simulink model "ball_and_plate_discreto2"  (Simulink 8.7)
settings: Solver=ode3  StartTime=0.0  StopTime=200  FixedStep=0.05  RelTol=1e-3
undefined symbols (not defined in the file): Newton, Raphson
settings Model: Creator=mario  LastModifiedBy=mario
settings DataIOCC: SaveFormat=Structure  SignalLoggingSaveFormat=ModelDataLogs
settings OptimizationCC: ExpressionDepthLimit=2147483647
settings DebuggingCC: SolverPrmCheckMsg=warning  FcnCallInpInsideContextMsg=UseLocalSettings  StateNameClashWarn=warning
settings GRTTargetCC: CombineOutputUpdateFcns=off  GRTInterface=on

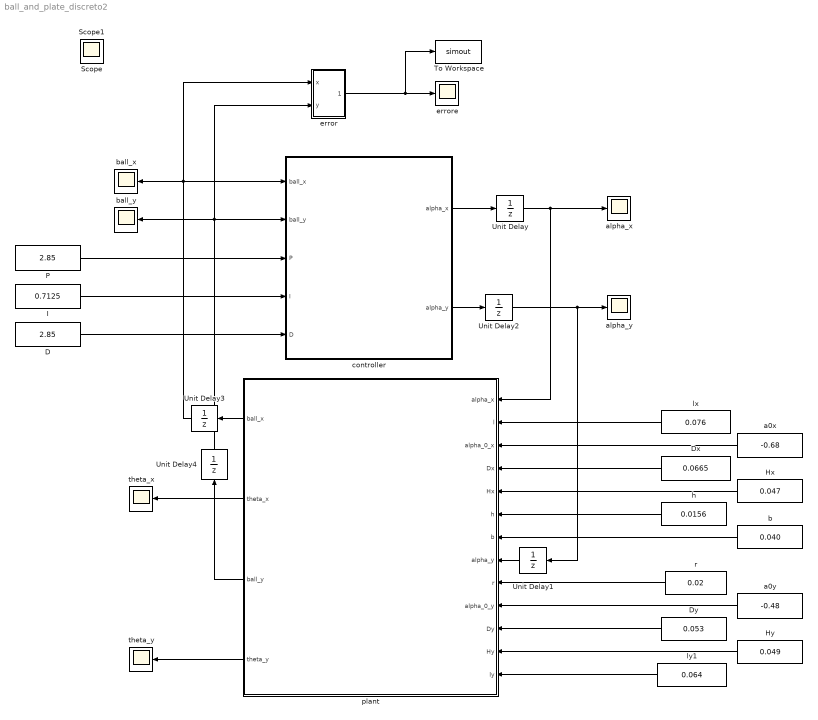
== system ball_and_plate_discreto2 ==
  D : Constant  Value=2.85  SampleTime=-1
  Dx : Constant  Value=0.0665
  Dy : Constant  Value=0.053
  Hx : Constant  Value=0.047
  Hy : Constant  Value=0.049
  I : Constant  Value=0.7125  SampleTime=-1
  P : Constant  Value=2.85  SampleTime=-1
  To Workspace : ToWorkspace  VariableName=simout  SampleTime=-1
  Unit Delay{,1..4} (5 alike) : UnitDelay  SampleTime=-1
  a0x : Constant  Value=-0.68  SampleTime=-1
  a0y : Constant  Value=-0.48  SampleTime=-1
  alpha_x : Scope
  alpha_y : Scope
  b : Constant  Value=0.040
  ball_x : Scope
  ball_y : Scope
  controller : Subsystem
  error : Subsystem
  errore : Scope
  h : Constant  Value=0.0156
  lx : Constant  Value=0.076
  ly1 : Constant  Value=0.064
  plant : Subsystem
  r : Constant  Value=0.02
  theta_x : Scope
  theta_y : Scope
  Scope : Scope
  Scope1 : Scope
  wires:
  error/1(error) -> errore/1, To Workspace/1
  plant/1(ball_x) -> Unit Delay3/1
  a0x/1 -> plant/3(alpha_0_x)
  Dx/1 -> plant/4(Dx)
  Hx/1 -> plant/5(Hx)
  plant/2(theta_x) -> theta_x/1
  controller/2(alpha_y) -> Unit Delay2/1
  a0y/1 -> plant/10(alpha_0_y)
  Dy/1 -> plant/11(Dy)
  Hy/1 -> plant/12(Hy)
  lx/1 -> plant/2(l)
  h/1 -> plant/6(h)
  b/1 -> plant/7(b)
  r/1 -> plant/9(r)
  plant/3(ball_y) -> Unit Delay4/1
  plant/4(theta_y) -> theta_y/1
  ly1/1 -> plant/13(ly)
  P/1 -> controller/3(P)
  I/1 -> controller/4(I)
  D/1 -> controller/5(D)
  controller/1(alpha_x) -> Unit Delay/1
  Unit Delay1/1 -> plant/8(alpha_y)
  Unit Delay/1 -> plant/1(alpha_x), alpha_x/1
  Unit Delay2/1 -> Unit Delay1/1, alpha_y/1
  Unit Delay3/1 -> controller/1(ball_x), ball_x/1, error/1(x)
  Unit Delay4/1 -> controller/2(ball_y), ball_y/1, error/2(y)

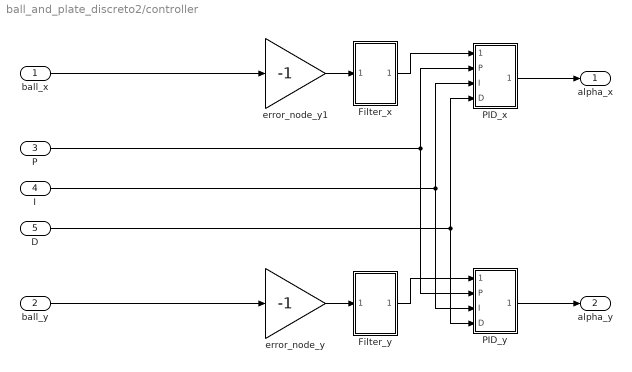
== system ball_and_plate_discreto2/controller ==
  ball_x : Inport
  ball_y : Inport  Port=2
  P : Inport  Port=3
  I : Inport  Port=4
  D : Inport  Port=5
  Filter_x : Subsystem
  Filter_y : Subsystem
  PID_x : Subsystem
  PID_y : Subsystem
  error_node_y : Gain  Gain=-1  SampleTime=50e-3
  error_node_y1 : Gain  Gain=-1  SampleTime=50e-3
  alpha_x : Outport
  alpha_y : Outport  Port=2
  wires:
  error_node_y1/1 -> Filter_x/1(In1)
  error_node_y/1 -> Filter_y/1(In1)
  Filter_y/1(Out1) -> PID_y/1(In1)
  ball_y/1 -> error_node_y/1
  ball_x/1 -> error_node_y1/1
  PID_y/1(Out1) -> alpha_y/1
  PID_x/1(Out1) -> alpha_x/1
  Filter_x/1(Out1) -> PID_x/1(In1)
  P/1 -> PID_x/2(P), PID_y/2(P)
  I/1 -> PID_x/3(I), PID_y/3(I)
  D/1 -> PID_x/4(D), PID_y/4(D)

== system ball_and_plate_discreto2/error ==
  x : Inport
  y : Inport  Port=2
  Product : Product  RndMeth=Zero
  Product1 : Product  RndMeth=Zero
  Sqrt : Sqrt  AlgorithmType=Newton-Raphson  SaturateOnIntegerOverflow=on
  Sum : Sum
  error : Outport
  wires:
  Sum/1 -> Sqrt/1
  Product1/1 -> Sum/1
  Product/1 -> Sum/2
  y/1 -> Product/2, Product/1
  x/1 -> Product1/1, Product1/2
  Sqrt/1 -> error/1

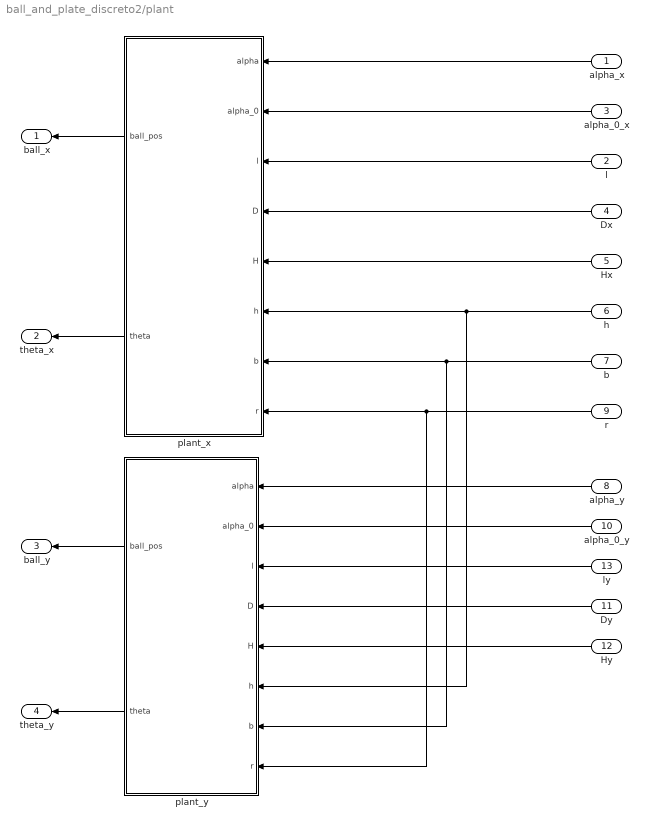
== system ball_and_plate_discreto2/plant ==
  alpha_x : Inport
  l : Inport  Port=2
  alpha_0_x : Inport  Port=3
  Dx : Inport  Port=4
  Hx : Inport  Port=5
  h : Inport  Port=6
  b : Inport  Port=7
  alpha_y : Inport  Port=8
  r : Inport  Port=9
  alpha_0_y : Inport  Port=10
  Dy : Inport  Port=11
  Hy : Inport  Port=12
  ly : Inport  Port=13
  plant_x : Subsystem
  plant_y : Subsystem
  ball_x : Outport
  theta_x : Outport  Port=2
  ball_y : Outport  Port=3
  theta_y : Outport  Port=4
  wires:
  l/1 -> plant_x/3(l)
  h/1 -> plant_y/6(h), plant_x/6(h)
  b/1 -> plant_y/7(b), plant_x/7(b)
  r/1 -> plant_y/8(r), plant_x/8(r)
  alpha_0_x/1 -> plant_x/2(alpha_0)
  plant_x/1(ball_pos) -> ball_x/1
  Dx/1 -> plant_x/4(D)
  Hx/1 -> plant_x/5(H)
  plant_x/2(theta) -> theta_x/1
  alpha_y/1 -> plant_y/1(alpha)
  alpha_0_y/1 -> plant_y/2(alpha_0)
  plant_y/1(ball_pos) -> ball_y/1
  Dy/1 -> plant_y/4(D)
  Hy/1 -> plant_y/5(H)
  plant_y/2(theta) -> theta_y/1
  ly/1 -> plant_y/3(l)
  alpha_x/1 -> plant_x/1(alpha)

== system ball_and_plate_discreto2/controller/Filter_x ==
  In1 : Inport
  Gain1 : Gain  Gain=0.714  SampleTime=50e-3
  Gain2 : Gain  Gain=-0.6  SampleTime=50e-3
  Integer Delay : Delay  DelayLength=1  InputProcessing=Inherited
  Integer Delay1 : Delay  DelayLength=1  InputProcessing=Inherited  SampleTime=50e-3
  Sum : Sum  Inputs=|+++  SampleTime=50e-3
  Out1 : Outport
  wires:
  Sum/1 -> Gain1/1
  Gain1/1 -> Integer Delay1/1, Out1/1
  Integer Delay1/1 -> Gain2/1
  Integer Delay/1 -> Sum/1
  Gain2/1 -> Sum/3
  In1/1 -> Integer Delay/1, Sum/2

== system ball_and_plate_discreto2/controller/Filter_y ==
  In1 : Inport
  Gain1 : Gain  Gain=0.714  SampleTime=50e-3
  Gain2 : Gain  Gain=-0.6  SampleTime=50e-3
  Integer Delay : Delay  DelayLength=1  InputProcessing=Inherited  SampleTime=50e-3
  Integer Delay1 : Delay  DelayLength=1  InputProcessing=Inherited  SampleTime=50e-3
  Sum : Sum  Inputs=+++  SampleTime=50e-3
  Out1 : Outport
  wires:
  Integer Delay1/1 -> Gain2/1
  Gain1/1 -> Integer Delay1/1, Out1/1
  Sum/1 -> Gain1/1
  Integer Delay/1 -> Sum/1
  In1/1 -> Integer Delay/1, Sum/2
  Gain2/1 -> Sum/3

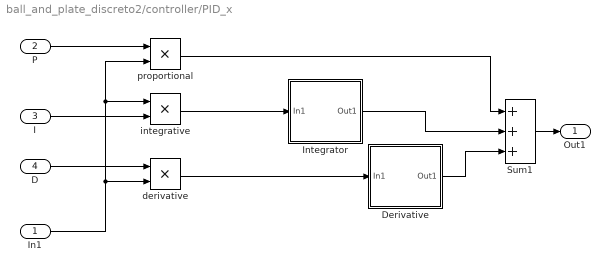
== system ball_and_plate_discreto2/controller/PID_x ==
  In1 : Inport
  P : Inport  Port=2
  I : Inport  Port=3
  D : Inport  Port=4
  Derivative : Subsystem
  Integrator : Subsystem
  Sum1 : Sum  Inputs=+++  SampleTime=50e-3
  derivative : Product  RndMeth=Zero
  integrative : Product  RndMeth=Zero
  proportional : Product  RndMeth=Zero
  Out1 : Outport
  wires:
  Sum1/1 -> Out1/1
  derivative/1 -> Derivative/1(In1)
  proportional/1 -> Sum1/1
  Integrator/1(Out1) -> Sum1/2
  Derivative/1(Out1) -> Sum1/3
  I/1 -> integrative/2
  D/1 -> derivative/1
  In1/1 -> proportional/2, integrative/1, derivative/2
  P/1 -> proportional/1
  integrative/1 -> Integrator/1(In1)

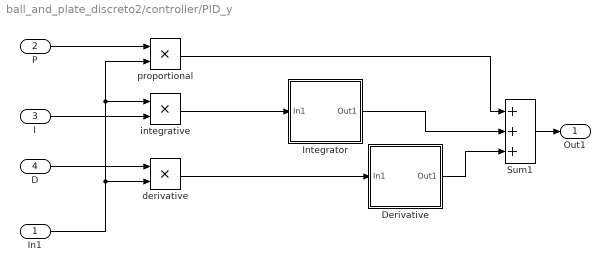
== system ball_and_plate_discreto2/controller/PID_y ==
  In1 : Inport
  P : Inport  Port=2
  I : Inport  Port=3
  D : Inport  Port=4
  Derivative : Subsystem
  Integrator : Subsystem
  Sum1 : Sum  Inputs=+++  SampleTime=50e-3
  derivative : Product  RndMeth=Zero
  integrative : Product  RndMeth=Zero
  proportional : Product  RndMeth=Zero
  Out1 : Outport
  wires:
  Sum1/1 -> Out1/1
  derivative/1 -> Derivative/1(In1)
  proportional/1 -> Sum1/1
  Integrator/1(Out1) -> Sum1/2
  Derivative/1(Out1) -> Sum1/3
  I/1 -> integrative/2
  D/1 -> derivative/1
  In1/1 -> proportional/2, integrative/1, derivative/2
  P/1 -> proportional/1
  integrative/1 -> Integrator/1(In1)

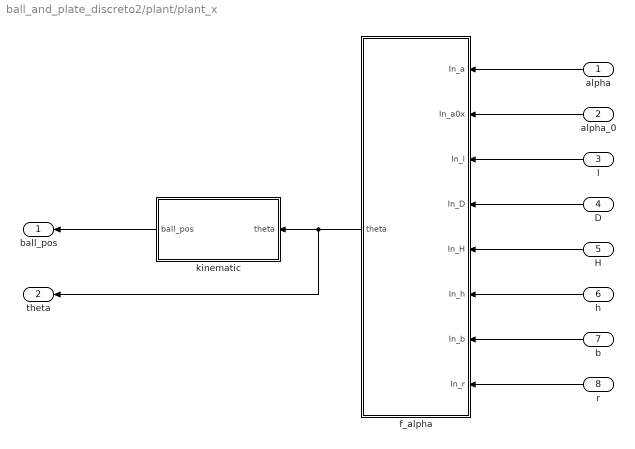
== system ball_and_plate_discreto2/plant/plant_x ==
  alpha : Inport
  alpha_0 : Inport  Port=2
  l : Inport  Port=3
  D : Inport  Port=4
  H : Inport  Port=5
  h : Inport  Port=6
  b : Inport  Port=7
  r : Inport  Port=8
  f_alpha : Subsystem
  kinematic : Subsystem
  ball_pos : Outport
  theta : Outport  Port=2
  wires:
  f_alpha/1(theta) -> theta/1, kinematic/1(theta)
  alpha/1 -> f_alpha/1(In_a)
  alpha_0/1 -> f_alpha/2(In_a0x)
  l/1 -> f_alpha/3(In_l)
  D/1 -> f_alpha/4(In_D)
  H/1 -> f_alpha/5(In_H)
  h/1 -> f_alpha/6(In_h)
  b/1 -> f_alpha/7(In_b)
  r/1 -> f_alpha/8(In_r)
  kinematic/1(ball_pos) -> ball_pos/1

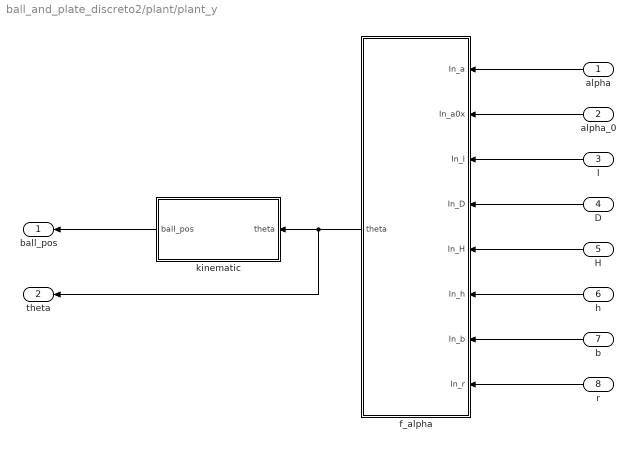
== system ball_and_plate_discreto2/plant/plant_y ==
  alpha : Inport
  alpha_0 : Inport  Port=2
  l : Inport  Port=3
  D : Inport  Port=4
  H : Inport  Port=5
  h : Inport  Port=6
  b : Inport  Port=7
  r : Inport  Port=8
  f_alpha : Subsystem
  kinematic : Subsystem
  ball_pos : Outport
  theta : Outport  Port=2
  wires:
  f_alpha/1(theta) -> theta/1, kinematic/1(theta)
  alpha/1 -> f_alpha/1(In_a)
  alpha_0/1 -> f_alpha/2(In_a0x)
  l/1 -> f_alpha/3(In_l)
  D/1 -> f_alpha/4(In_D)
  H/1 -> f_alpha/5(In_H)
  h/1 -> f_alpha/6(In_h)
  b/1 -> f_alpha/7(In_b)
  r/1 -> f_alpha/8(In_r)
  kinematic/1(ball_pos) -> ball_pos/1

== system ball_and_plate_discreto2/controller/PID_x/Derivative ==
  In1 : Inport
  Gain3 : Gain  Gain=20  SampleTime=50e-3
  Integer Delay1 : Delay  DelayLength=1  InputProcessing=Inherited  SampleTime=50e-3
  Sum : Sum  Inputs=|+-
  Out1 : Outport
  wires:
  Gain3/1 -> Out1/1
  In1/1 -> Sum/1, Integer Delay1/1
  Sum/1 -> Gain3/1
  Integer Delay1/1 -> Sum/2

== system ball_and_plate_discreto2/controller/PID_x/Integrator ==
  In1 : Inport
  Gain1 : Gain  Gain=50e-3  SampleTime=50e-3
  Integer Delay : Delay  DelayLength=1  InputProcessing=Inherited  SampleTime=50e-3
  Integer Delay1 : Delay  DelayLength=1  InputProcessing=Inherited  SampleTime=50e-3
  Sum : Sum  Inputs=|++
  Out1 : Outport
  wires:
  Gain1/1 -> Sum/1
  Integer Delay/1 -> Gain1/1
  Sum/1 -> Integer Delay1/1, Out1/1
  In1/1 -> Integer Delay/1
  Integer Delay1/1 -> Sum/2

== system ball_and_plate_discreto2/controller/PID_y/Derivative ==
  In1 : Inport
  Gain3 : Gain  Gain=20  SampleTime=50e-3
  Integer Delay1 : Delay  DelayLength=1  InputProcessing=Inherited  SampleTime=50e-3
  Sum : Sum  Inputs=|+-
  Out1 : Outport
  wires:
  Gain3/1 -> Out1/1
  In1/1 -> Sum/1, Integer Delay1/1
  Sum/1 -> Gain3/1
  Integer Delay1/1 -> Sum/2

== system ball_and_plate_discreto2/controller/PID_y/Integrator ==
  In1 : Inport
  Gain1 : Gain  Gain=50e-3  SampleTime=50e-3
  Integer Delay : Delay  DelayLength=1  InputProcessing=Inherited  SampleTime=50e-3
  Integer Delay1 : Delay  DelayLength=1  InputProcessing=Inherited  SampleTime=50e-3
  Sum : Sum  Inputs=|++
  Out1 : Outport
  wires:
  Gain1/1 -> Sum/1
  Integer Delay/1 -> Gain1/1
  Sum/1 -> Integer Delay1/1, Out1/1
  In1/1 -> Integer Delay/1
  Integer Delay1/1 -> Sum/2

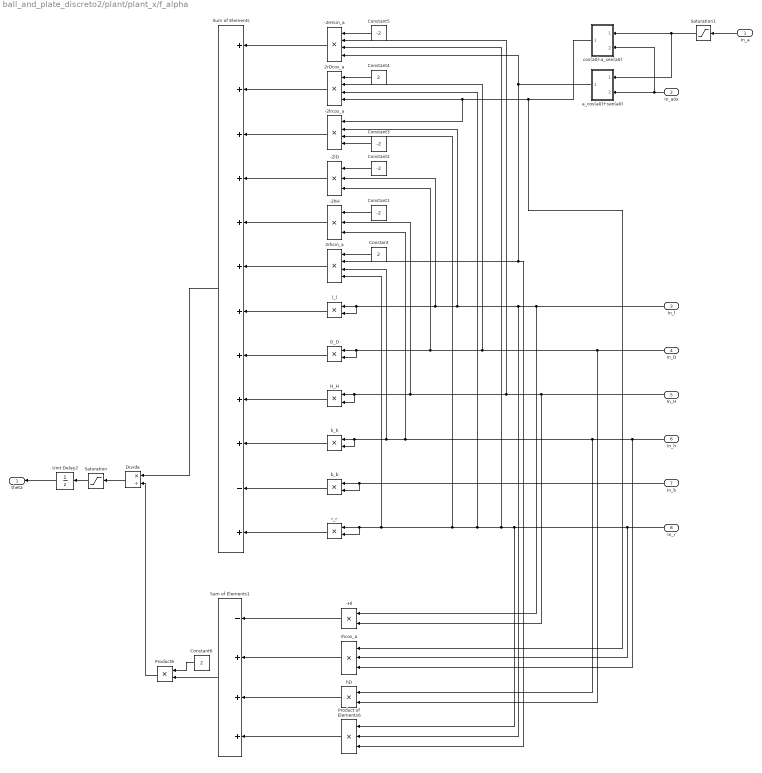
== system ball_and_plate_discreto2/plant/plant_x/f_alpha ==
  In_a : Inport
  In_a0x : Inport  Port=2
  In_l : Inport  Port=3
  In_D : Inport  Port=4
  In_H : Inport  Port=5
  In_h : Inport  Port=6
  In_b : Inport  Port=7
  In_r : Inport  Port=8
  -2Hrsin_a : Product  Inputs=4
  -2hH : Product  Inputs=3
  -2lD : Product  Inputs=3
  -2lrcos_a : Product  Inputs=4
  -Hl : Product
  2rDcos_a : Product  Inputs=4
  2rhsin_a : Product  Inputs=4
  Constant : Constant  Value=2
  Constant1 : Constant  Value=-2
  Constant2 : Constant  Value=-2  SampleTime=0.05
  Constant3 : Constant  Value=-2  SampleTime=0.05
  Constant4 : Constant  Value=2
  Constant5 : Constant  Value=-2
  Constant6 : Constant  Value=2
  D_D : Product  RndMeth=Zero
  Divide : Product  Inputs=*/
  H_H : Product  RndMeth=Zero
  Product of Elements6 : Product  Inputs=3  SampleTime=0.05
  Product6 : Product  RndMeth=Zero
  Saturation : Saturate  UpperLimit=0.05  LowerLimit=-0.05
  Saturation1 : Saturate
  Sum of Elements : Sum  Inputs=++++++++++-+
  Sum of Elements1 : Sum  Inputs=-+++
  Unit Delay2 : UnitDelay  SampleTime=-1
  a_cos(a0)+sen(a0) : Subsystem
  b_b : Product  RndMeth=Zero
  cos(a0)-a_sen(a0) : Subsystem
  hD : Product
  h_h : Product  RndMeth=Zero
  l_l : Product  RndMeth=Zero
  r_r : Product  RndMeth=Zero
  rhcos_a : Product  Inputs=3
  theta : Outport
  wires:
  In_H/1 -> -Hl/2, -2Hrsin_a/2, -2hH/2, H_H/1, H_H/2
  In_r/1 -> rhcos_a/2, Product of Elements6/1, -2Hrsin_a/3, 2rDcos_a/3, -2lrcos_a/3, 2rhsin_a/4, r_r/1, r_r/2
  In_h/1 -> hD/1, -2hH/3, 2rhsin_a/3, h_h/1, h_h/2, rhcos_a/3
  In_b/1 -> b_b/1, b_b/2
  In_a0x/1 -> cos(a0)-a_sen(a0)/2(In2), a_cos(a0)+sen(a0)/2(In2)
  r_r/1 -> Sum of Elements/12
  b_b/1 -> Sum of Elements/11
  h_h/1 -> Sum of Elements/10
  H_H/1 -> Sum of Elements/9
  D_D/1 -> Sum of Elements/8
  In_D/1 -> hD/2, 2rDcos_a/2, -2lD/3, D_D/2, D_D/1
  In_l/1 -> -Hl/1, Product of Elements6/2, -2lrcos_a/2, -2lD/2, l_l/2, l_l/1
  l_l/1 -> Sum of Elements/7
  Constant/1 -> 2rhsin_a/1
  a_cos(a0)+sen(a0)/1(Out1) -> -2Hrsin_a/4, 2rhsin_a/2, Product of Elements6/3
  2rhsin_a/1 -> Sum of Elements/6
  Constant1/1 -> -2hH/1
  -2hH/1 -> Sum of Elements/5
  Constant2/1 -> -2lD/1
  Constant3/1 -> -2lrcos_a/4
  cos(a0)-a_sen(a0)/1(Out1) -> -2lrcos_a/1, 2rDcos_a/4, rhcos_a/1
  -2lD/1 -> Sum of Elements/4
  -2lrcos_a/1 -> Sum of Elements/3
  Constant4/1 -> 2rDcos_a/1
  2rDcos_a/1 -> Sum of Elements/2
  Constant5/1 -> -2Hrsin_a/1
  -2Hrsin_a/1 -> Sum of Elements/1
  Product of Elements6/1 -> Sum of Elements1/4
  hD/1 -> Sum of Elements1/3
  rhcos_a/1 -> Sum of Elements1/2
  -Hl/1 -> Sum of Elements1/1
  Sum of Elements1/1 -> Product6/2
  Constant6/1 -> Product6/1
  Sum of Elements/1 -> Divide/1
  Product6/1 -> Divide/2
  In_a/1 -> Saturation1/1
  Divide/1 -> Saturation/1
  Saturation1/1 -> cos(a0)-a_sen(a0)/1(In1), a_cos(a0)+sen(a0)/1(In1)
  Saturation/1 -> Unit Delay2/1
  Unit Delay2/1 -> theta/1

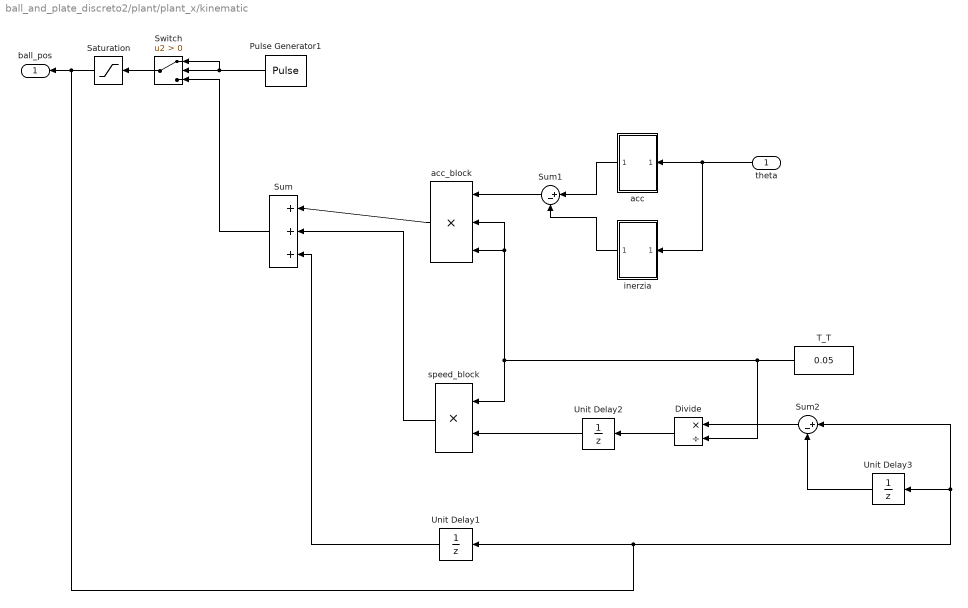
== system ball_and_plate_discreto2/plant/plant_x/kinematic ==
  theta : Inport
  Divide : Product  Inputs=*/
  Pulse Generator1 : DiscretePulseGenerator  Amplitude=0.0704  Period=4800  PhaseDelay=400  SampleTime=0.05
  Saturation : Saturate  UpperLimit=0.0704  LowerLimit=-0.0704
  Sum : Sum  Inputs=|+++
  Sum1 : Sum  Inputs=|+-
  Sum2 : Sum  Inputs=|+-
  Switch : Switch  Criteria=u2 > Threshold
  T_T : Constant  Value=0.05  SampleTime=0.05
  Unit Delay1 : UnitDelay  SampleTime=0.05
  Unit Delay2 : UnitDelay  SampleTime=0.05
  Unit Delay3 : UnitDelay  SampleTime=0.05
  acc : Subsystem
  acc_block : Product  Inputs=3  RndMeth=Zero
  inerzia : Subsystem
  speed_block : Product  RndMeth=Zero
  ball_pos : Outport
  wires:
  Pulse Generator1/1 -> Switch/1, Switch/2
  Sum/1 -> Switch/3
  Unit Delay2/1 -> speed_block/2
  Unit Delay3/1 -> Sum2/2
  Sum2/1 -> Divide/1
  Divide/1 -> Unit Delay2/1
  acc/1(Out1) -> Sum1/1
  Switch/1 -> Saturation/1
  Saturation/1 -> Unit Delay3/1, Sum2/1, Unit Delay1/1, ball_pos/1
  inerzia/1(Out1) -> Sum1/2
  acc_block/1 -> Sum/1
  speed_block/1 -> Sum/2
  Unit Delay1/1 -> Sum/3
  Sum1/1 -> acc_block/1
  theta/1 -> acc/1(In1), inerzia/1(In1)
  T_T/1 -> speed_block/1, acc_block/3, acc_block/2, Divide/2

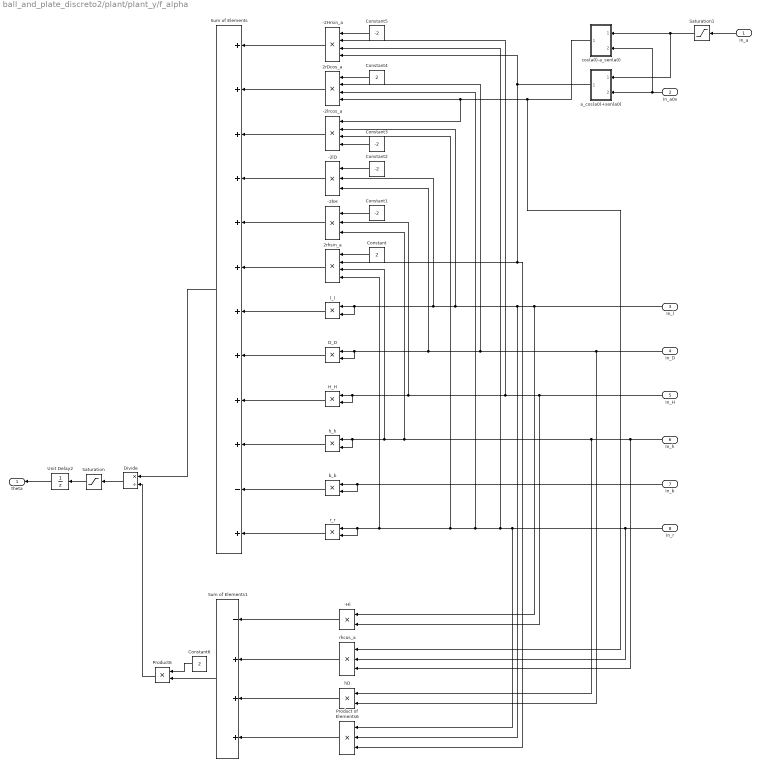
== system ball_and_plate_discreto2/plant/plant_y/f_alpha ==
  In_a : Inport
  In_a0x : Inport  Port=2
  In_l : Inport  Port=3
  In_D : Inport  Port=4
  In_H : Inport  Port=5
  In_h : Inport  Port=6
  In_b : Inport  Port=7
  In_r : Inport  Port=8
  -2Hrsin_a : Product  Inputs=4
  -2hH : Product  Inputs=3
  -2lD : Product  Inputs=3
  -2lrcos_a : Product  Inputs=4
  -Hl : Product
  2rDcos_a : Product  Inputs=4
  2rhsin_a : Product  Inputs=4
  Constant : Constant  Value=2
  Constant1 : Constant  Value=-2
  Constant2 : Constant  Value=-2  SampleTime=0.05
  Constant3 : Constant  Value=-2  SampleTime=0.05
  Constant4 : Constant  Value=2
  Constant5 : Constant  Value=-2
  Constant6 : Constant  Value=2
  D_D : Product  RndMeth=Zero
  Divide : Product  Inputs=*/
  H_H : Product  RndMeth=Zero
  Product of Elements6 : Product  Inputs=3  SampleTime=0.05
  Product6 : Product  RndMeth=Zero
  Saturation : Saturate  UpperLimit=0.2  LowerLimit=-0.2
  Saturation1 : Saturate
  Sum of Elements : Sum  Inputs=++++++++++-+
  Sum of Elements1 : Sum  Inputs=-+++
  Unit Delay2 : UnitDelay  SampleTime=-1
  a_cos(a0)+sen(a0) : Subsystem
  b_b : Product  RndMeth=Zero
  cos(a0)-a_sen(a0) : Subsystem
  hD : Product
  h_h : Product  RndMeth=Zero
  l_l : Product  RndMeth=Zero
  r_r : Product  RndMeth=Zero
  rhcos_a : Product  Inputs=3
  theta : Outport
  wires:
  In_H/1 -> -Hl/2, -2Hrsin_a/2, -2hH/2, H_H/1, H_H/2
  In_r/1 -> rhcos_a/2, Product of Elements6/1, -2Hrsin_a/3, 2rDcos_a/3, -2lrcos_a/3, 2rhsin_a/4, r_r/1, r_r/2
  In_h/1 -> hD/1, -2hH/3, 2rhsin_a/3, h_h/1, h_h/2, rhcos_a/3
  In_b/1 -> b_b/1, b_b/2
  In_a0x/1 -> cos(a0)-a_sen(a0)/2(In2), a_cos(a0)+sen(a0)/2(In2)
  r_r/1 -> Sum of Elements/12
  b_b/1 -> Sum of Elements/11
  h_h/1 -> Sum of Elements/10
  H_H/1 -> Sum of Elements/9
  D_D/1 -> Sum of Elements/8
  In_D/1 -> hD/2, 2rDcos_a/2, -2lD/3, D_D/2, D_D/1
  In_l/1 -> -Hl/1, Product of Elements6/2, -2lrcos_a/2, -2lD/2, l_l/2, l_l/1
  l_l/1 -> Sum of Elements/7
  Constant/1 -> 2rhsin_a/1
  a_cos(a0)+sen(a0)/1(Out1) -> -2Hrsin_a/4, 2rhsin_a/2, Product of Elements6/3
  2rhsin_a/1 -> Sum of Elements/6
  Constant1/1 -> -2hH/1
  -2hH/1 -> Sum of Elements/5
  Constant2/1 -> -2lD/1
  Constant3/1 -> -2lrcos_a/4
  cos(a0)-a_sen(a0)/1(Out1) -> -2lrcos_a/1, 2rDcos_a/4, rhcos_a/1
  -2lD/1 -> Sum of Elements/4
  -2lrcos_a/1 -> Sum of Elements/3
  Constant4/1 -> 2rDcos_a/1
  2rDcos_a/1 -> Sum of Elements/2
  Constant5/1 -> -2Hrsin_a/1
  -2Hrsin_a/1 -> Sum of Elements/1
  Product of Elements6/1 -> Sum of Elements1/4
  hD/1 -> Sum of Elements1/3
  rhcos_a/1 -> Sum of Elements1/2
  -Hl/1 -> Sum of Elements1/1
  Sum of Elements1/1 -> Product6/2
  Constant6/1 -> Product6/1
  Sum of Elements/1 -> Divide/1
  Product6/1 -> Divide/2
  In_a/1 -> Saturation1/1
  Divide/1 -> Saturation/1
  Saturation/1 -> Unit Delay2/1
  Saturation1/1 -> cos(a0)-a_sen(a0)/1(In1), a_cos(a0)+sen(a0)/1(In1)
  Unit Delay2/1 -> theta/1

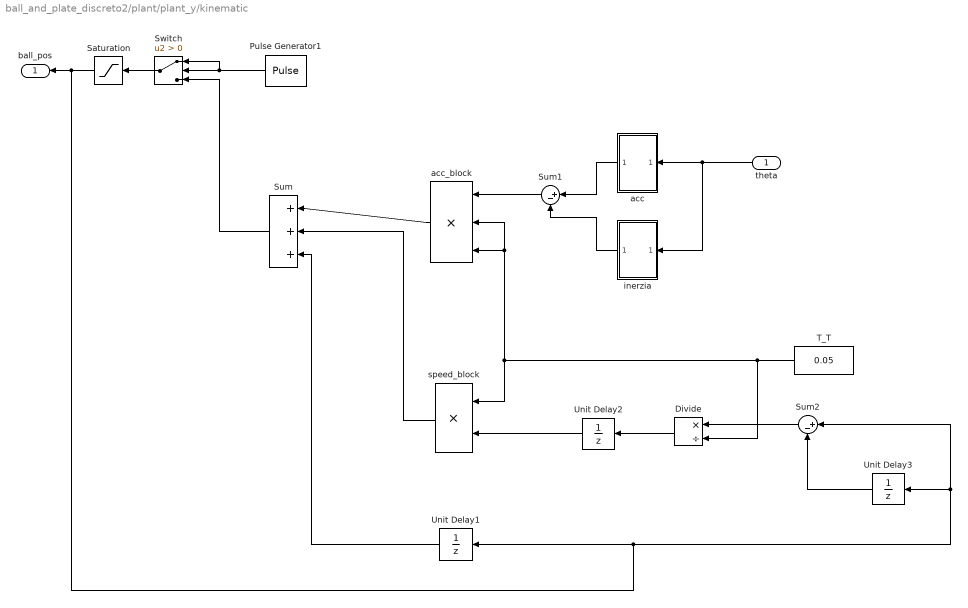
== system ball_and_plate_discreto2/plant/plant_y/kinematic ==
  theta : Inport
  Divide : Product  Inputs=*/
  Pulse Generator1 : DiscretePulseGenerator  Amplitude=0.097  Period=4800  PhaseDelay=400  SampleTime=0.05
  Saturation : Saturate  UpperLimit=0.097  LowerLimit=-0.097
  Sum : Sum  Inputs=|+++
  Sum1 : Sum  Inputs=|+-
  Sum2 : Sum  Inputs=|+-
  Switch : Switch  Criteria=u2 > Threshold
  T_T : Constant  Value=0.05  SampleTime=0.05
  Unit Delay1 : UnitDelay  SampleTime=0.05
  Unit Delay2 : UnitDelay  SampleTime=0.05
  Unit Delay3 : UnitDelay  SampleTime=0.05
  acc : Subsystem
  acc_block : Product  Inputs=3  RndMeth=Zero
  inerzia : Subsystem
  speed_block : Product  RndMeth=Zero
  ball_pos : Outport
  wires:
  Pulse Generator1/1 -> Switch/1, Switch/2
  Sum/1 -> Switch/3
  Unit Delay2/1 -> speed_block/2
  Unit Delay3/1 -> Sum2/2
  Sum2/1 -> Divide/1
  Divide/1 -> Unit Delay2/1
  acc/1(Out1) -> Sum1/1
  Switch/1 -> Saturation/1
  Saturation/1 -> Unit Delay3/1, Sum2/1, Unit Delay1/1, ball_pos/1
  inerzia/1(Out1) -> Sum1/2
  acc_block/1 -> Sum/1
  speed_block/1 -> Sum/2
  Unit Delay1/1 -> Sum/3
  Sum1/1 -> acc_block/1
  theta/1 -> acc/1(In1), inerzia/1(In1)
  T_T/1 -> acc_block/3, acc_block/2, speed_block/1, Divide/2

== system ball_and_plate_discreto2/plant/plant_x/f_alpha/a_cos(a0)+sen(a0) ==
  In1 : Inport
  In2 : Inport  Port=2
  Product6 : Product  RndMeth=Zero
  Sum : Sum  Inputs=|++
  Trigonometric Function : Trigonometry  Operator=cos
  Trigonometric Function1 : Trigonometry
  Out1 : Outport
  wires:
  Trigonometric Function/1 -> Product6/2
  Product6/1 -> Sum/1
  Trigonometric Function1/1 -> Sum/2
  In2/1 -> Trigonometric Function/1, Trigonometric Function1/1
  Sum/1 -> Out1/1
  In1/1 -> Product6/1

== system ball_and_plate_discreto2/plant/plant_x/f_alpha/cos(a0)-a_sen(a0) ==
  In1 : Inport
  In2 : Inport  Port=2
  Product6 : Product  RndMeth=Zero
  Sum : Sum  Inputs=|-+
  Trigonometric Function : Trigonometry
  Trigonometric Function1 : Trigonometry  Operator=cos
  Out1 : Outport
  wires:
  Trigonometric Function/1 -> Product6/2
  Product6/1 -> Sum/1
  Trigonometric Function1/1 -> Sum/2
  In2/1 -> Trigonometric Function1/1, Trigonometric Function/1
  Sum/1 -> Out1/1
  In1/1 -> Product6/1

== system ball_and_plate_discreto2/plant/plant_x/kinematic/acc ==
  In1 : Inport
  Product of Elements : Product
  Scope : Scope
  Trigonometric Function : Trigonometry
  alpha : Subsystem
  Out1 : Outport
  wires:
  Trigonometric Function/1 -> Product of Elements/1
  In1/1 -> Trigonometric Function/1
  Product of Elements/1 -> Out1/1, Scope/1
  alpha/1(Out1) -> Product of Elements/2

== system ball_and_plate_discreto2/plant/plant_x/kinematic/inerzia ==
  In1 : Inport
  Divide2 : Product  Inputs=*/
  Product of Elements1 : Product
  Subsystem : Subsystem
  Subsystem1 : Subsystem
  Subtract3 : Sum  Inputs=+-
  T1 : Constant  Value=0.05  VectorParams1D=off  SampleTime=0.05
  beta : Constant  Value=0.054  VectorParams1D=off  SampleTime=0.05
  Out1 : Outport
  wires:
  Subtract3/1 -> Divide2/1
  T1/1 -> Divide2/2
  Subsystem1/1(Out1) -> Subtract3/2
  Product of Elements1/1 -> Out1/1
  Divide2/1 -> Product of Elements1/1
  beta/1 -> Product of Elements1/2
  Subsystem/1(Out1) -> Subtract3/1
  In1/1 -> Subsystem/1(In1), Subsystem1/1(In1)

== system ball_and_plate_discreto2/plant/plant_y/f_alpha/a_cos(a0)+sen(a0) ==
  In1 : Inport
  In2 : Inport  Port=2
  Product6 : Product  RndMeth=Zero
  Sum : Sum  Inputs=|++
  Trigonometric Function : Trigonometry  Operator=cos
  Trigonometric Function1 : Trigonometry
  Out1 : Outport
  wires:
  Trigonometric Function/1 -> Product6/2
  Product6/1 -> Sum/1
  Trigonometric Function1/1 -> Sum/2
  In2/1 -> Trigonometric Function/1, Trigonometric Function1/1
  Sum/1 -> Out1/1
  In1/1 -> Product6/1

== system ball_and_plate_discreto2/plant/plant_y/f_alpha/cos(a0)-a_sen(a0) ==
  In1 : Inport
  In2 : Inport  Port=2
  Product6 : Product  RndMeth=Zero
  Sum : Sum  Inputs=|-+
  Trigonometric Function : Trigonometry
  Trigonometric Function1 : Trigonometry  Operator=cos
  Out1 : Outport
  wires:
  Trigonometric Function/1 -> Product6/2
  Product6/1 -> Sum/1
  Trigonometric Function1/1 -> Sum/2
  In2/1 -> Trigonometric Function1/1, Trigonometric Function/1
  Sum/1 -> Out1/1
  In1/1 -> Product6/1

== system ball_and_plate_discreto2/plant/plant_y/kinematic/acc ==
  In1 : Inport
  Product of Elements : Product
  Scope : Scope
  Trigonometric Function : Trigonometry
  alpha : Subsystem
  Out1 : Outport
  wires:
  Trigonometric Function/1 -> Product of Elements/1
  In1/1 -> Trigonometric Function/1
  Product of Elements/1 -> Out1/1, Scope/1
  alpha/1(Out1) -> Product of Elements/2

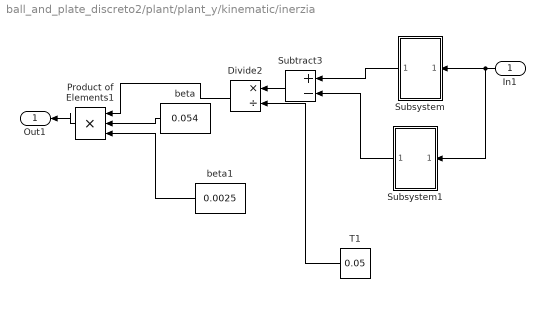
== system ball_and_plate_discreto2/plant/plant_y/kinematic/inerzia ==
  In1 : Inport
  Divide2 : Product  Inputs=*/
  Product of Elements1 : Product  Inputs=3
  Subsystem : Subsystem
  Subsystem1 : Subsystem
  Subtract3 : Sum  Inputs=+-
  T1 : Constant  Value=0.05  VectorParams1D=off  SampleTime=0.05
  beta : Constant  Value=0.054  VectorParams1D=off  SampleTime=0.05
  beta1 : Constant  Value=0.0025  VectorParams1D=off  SampleTime=0.05
  Out1 : Outport
  wires:
  Subsystem/1(Out1) -> Subtract3/1
  Subtract3/1 -> Divide2/1
  T1/1 -> Divide2/2
  Subsystem1/1(Out1) -> Subtract3/2
  In1/1 -> Subsystem/1(In1), Subsystem1/1(In1)
  Product of Elements1/1 -> Out1/1
  Divide2/1 -> Product of Elements1/1
  beta/1 -> Product of Elements1/2
  beta1/1 -> Product of Elements1/3

== system ball_and_plate_discreto2/plant/plant_x/kinematic/acc/alpha ==
  Divide1 : Product  Inputs=*/  SampleTime=0.05
  Product of Elements2 : Product
  g : Constant  Value=9.81  VectorParams1D=off  OutDataTypeStr=double  SampleTime=0.05
  inerzia_den : Constant  Value=7.0  VectorParams1D=off  OutDataTypeStr=double  SampleTime=0.05
  inerzia_num : Constant  Value=5.0  VectorParams1D=off  OutDataTypeStr=double  SampleTime=0.05
  Out1 : Outport
  wires:
  inerzia_num/1 -> Divide1/1
  inerzia_den/1 -> Divide1/2
  Product of Elements2/1 -> Out1/1
  g/1 -> Product of Elements2/1
  Divide1/1 -> Product of Elements2/2

== system ball_and_plate_discreto2/plant/plant_x/kinematic/inerzia/Subsystem ==
  In1 : Inport
  Divide : Product  Inputs=*/
  Subtract : Sum  Inputs=+-  SampleTime=0.05
  T1 : Constant  Value=0.05  VectorParams1D=off  SampleTime=0.05
  Unit Delay : UnitDelay  InitialCondition=-0.70  SampleTime=-1
  Out1 : Outport
  wires:
  Subtract/1 -> Divide/1
  T1/1 -> Divide/2
  Unit Delay/1 -> Subtract/2
  In1/1 -> Unit Delay/1, Subtract/1
  Divide/1 -> Out1/1

== system ball_and_plate_discreto2/plant/plant_x/kinematic/inerzia/Subsystem1 ==
  In1 : Inport
  Divide1 : Product  Inputs=*/
  Subtract1 : Sum  Inputs=+-  SampleTime=0.05
  T1 : Constant  Value=0.05  VectorParams1D=off  SampleTime=0.05
  Unit Delay1 : UnitDelay  InitialCondition=-0.7  SampleTime=0.05
  Unit Delay2 : UnitDelay  InitialCondition=-0.7  SampleTime=0.05
  Out1 : Outport
  wires:
  Unit Delay2/1 -> Unit Delay1/1, Subtract1/1
  Unit Delay1/1 -> Subtract1/2
  T1/1 -> Divide1/2
  Subtract1/1 -> Divide1/1
  Divide1/1 -> Out1/1
  In1/1 -> Unit Delay2/1

== system ball_and_plate_discreto2/plant/plant_y/kinematic/acc/alpha ==
  Divide1 : Product  Inputs=*/  SampleTime=0.05
  Product of Elements2 : Product
  g : Constant  Value=9.81  VectorParams1D=off  OutDataTypeStr=double  SampleTime=0.05
  inerzia_den : Constant  Value=7.0  VectorParams1D=off  OutDataTypeStr=double  SampleTime=0.05
  inerzia_num : Constant  Value=5.0  VectorParams1D=off  OutDataTypeStr=double  SampleTime=0.05
  Out1 : Outport
  wires:
  inerzia_num/1 -> Divide1/1
  inerzia_den/1 -> Divide1/2
  Product of Elements2/1 -> Out1/1
  g/1 -> Product of Elements2/1
  Divide1/1 -> Product of Elements2/2

== system ball_and_plate_discreto2/plant/plant_y/kinematic/inerzia/Subsystem ==
  In1 : Inport
  Divide : Product  Inputs=*/
  Subtract : Sum  Inputs=+-  SampleTime=0.05
  T1 : Constant  Value=0.05  VectorParams1D=off  SampleTime=0.05
  Unit Delay : UnitDelay  InitialCondition=-0.7  SampleTime=-1
  Out1 : Outport
  wires:
  Subtract/1 -> Divide/1
  T1/1 -> Divide/2
  Unit Delay/1 -> Subtract/2
  In1/1 -> Unit Delay/1, Subtract/1
  Divide/1 -> Out1/1

== system ball_and_plate_discreto2/plant/plant_y/kinematic/inerzia/Subsystem1 ==
  In1 : Inport
  Divide1 : Product  Inputs=*/
  Subtract1 : Sum  Inputs=+-  SampleTime=0.05
  T1 : Constant  Value=0.05  VectorParams1D=off  SampleTime=0.05
  Unit Delay1 : UnitDelay  InitialCondition=-0.7  SampleTime=0.05
  Unit Delay2 : UnitDelay  InitialCondition=-0.7  SampleTime=0.05
  Out1 : Outport
  wires:
  Unit Delay2/1 -> Unit Delay1/1, Subtract1/1
  Unit Delay1/1 -> Subtract1/2
  T1/1 -> Divide1/2
  Subtract1/1 -> Divide1/1
  Divide1/1 -> Out1/1
  In1/1 -> Unit Delay2/1
